simulink model "Pure_Pursuit_carsim"  (R2026a)
settings: Solver=FixedStepAuto  StopTime=15  FixedStep=0.0005
model workspace (MAT data in the model file):
  A = [0  1  20  0; 0  -6.22788393489  0  -17.6716206653; 0  0  0  1; 0  2.14095138934  0  -12.8986399427]
  B = [0; 65.1096956829; 0; 60.7665777315]
  C = [1  0  0  0; 0  1  0  0; 0  0  1  0; 0  0  0  1]
  Caf = 92000
  Car = 84000
  D = [0; 0; 0; 0]
  Iz = 1536.7
  Kd = 0.33
  Kp = 1
  N = 100
  T_delay = 0
  l_tot = 2.91
  la = 1.015
  lb = 1.895
  m = 1413
  u0 = 20
libraries: Solver_SF x1
settings Model: Creator=howardchueh  LastModifiedBy=Amy Lin
settings DataIOCC: SaveState=on

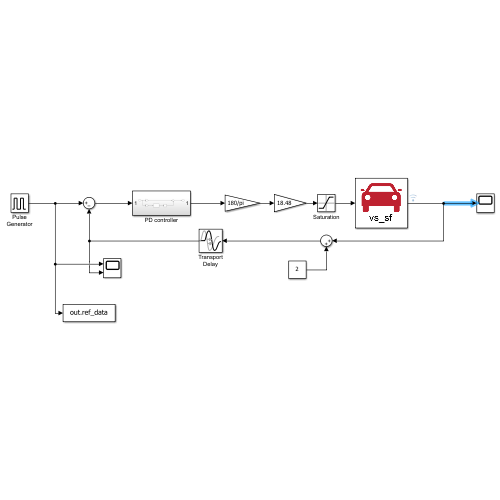
[thumbnail: Simulink's stored preview of the top-level diagram]
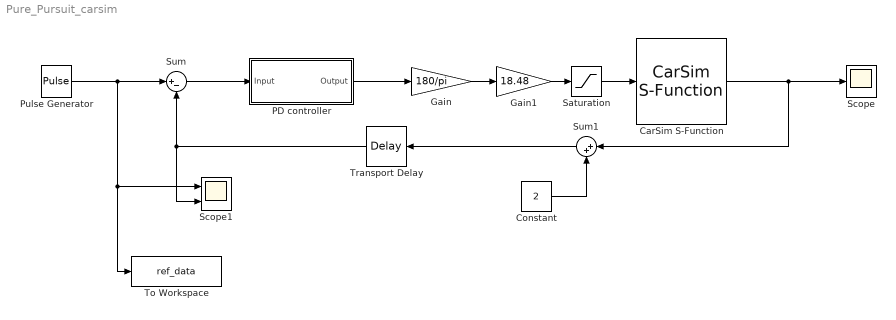
== system Pure_Pursuit_carsim ==
  CarSim S-Function : Solver_SF/CarSim S-Function  Priority=1  SIMFILE=simfile.sim  Run_RTs=off  vs_state_ind=Run  StopMode_ind=Vehicle Model
  Constant : Constant  Value=2
  Gain : Gain  Gain=180/pi
  Gain1 : Gain  Gain=18.48
  PD controller : Subsystem
  Pulse Generator : DiscretePulseGenerator  PulseType=Time based  Amplitude=4  Period=7  PulseWidth=50  PhaseDelay=0.5
  Saturation : Saturate  UpperLimit=48.7  LowerLimit=-48.7
  Scope : Scope
      settings: ActiveDisplayYMinimum=-4.0616664856018163  ActiveDisplayYMaximum=4.0607058814134787
  Scope1 : Scope  NumInputPorts=2
      settings: ActiveDisplayYMinimum=-1  ActiveDisplayYMaximum=1
  Sum : Sum  Inputs=|+-
  Sum1 : Sum  Inputs=|++
  To Workspace : ToWorkspace  VariableName=ref_data  SampleTime=-1
  Transport Delay : TransportDelay  DelayTime=T_delay
  wires:
  Pulse Generator/1 -> To Workspace/1, Scope1/1, Sum/1
  Sum/1 -> PD controller/1(Input)
  PD controller/1(Output) -> Gain/1
  Saturation/1 -> CarSim S-Function/1
  Transport Delay/1 -> Sum/2, Scope1/2
  Gain/1 -> Gain1/1
  Gain1/1 -> Saturation/1
  CarSim S-Function/1 -> Sum1/1, Scope/1
  Constant/1 -> Sum1/2
  Sum1/1 -> Transport Delay/1

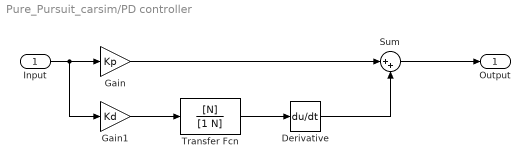
== system Pure_Pursuit_carsim/PD controller ==
  Input : Inport
  Derivative : Derivative
  Gain : Gain  Gain=Kp
  Gain1 : Gain  Gain=Kd
  Sum : Sum  Inputs=|++
  Transfer Fcn : TransferFcn  Numerator=[N]  Denominator=[1 N]
  Output : Outport
  wires:
  Gain1/1 -> Transfer Fcn/1
  Transfer Fcn/1 -> Derivative/1
  Gain/1 -> Sum/1
  Input/1 -> Gain1/1, Gain/1
  Derivative/1 -> Sum/2
  Sum/1 -> Output/1
